simulink model "VehicleLongitudnalModel"  (R2022a)
settings: Solver=FixedStepAuto  StartTime=4192  StopTime=max(time)  FixedStep=0.01  RelTol=1e-3
values from neighbouring files (symbols this model uses):
  g = 9.81    [ModelScript.m]
  ratio_fd = ratio_fd.*0.95    [ModelScript.m]
  vehMass = 2512    [ModelScript.m]
  vehMaxPower = 400e3    (= 400000)    [ModelScript.m]
  vehTireRadius = 0.5    [ModelScript.m]
libraries: slpidlib x1
settings Model: PacingRate=0.180000  Creator=saumi  LastModifiedBy=saumilj
settings DebuggingCC: AlgebraicLoopMsg=error  ArtificialAlgebraicLoopMsg=error
settings SFSimCC: SimTargetLang=C++

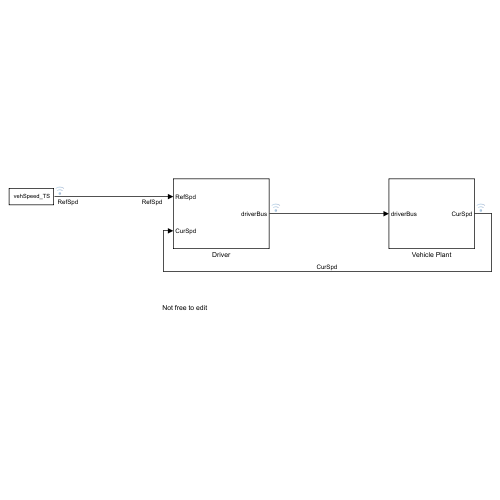
[thumbnail: Simulink's stored preview of the top-level diagram]
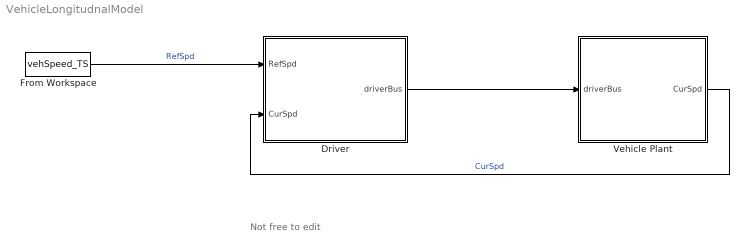
== system VehicleLongitudnalModel ==
  note: Not free to edit
  Driver : Subsystem
  From Workspace : FromWorkspace  VariableName=vehSpeed_TS
  Vehicle Plant : Subsystem
  wires:
  From Workspace/1 -> Driver/1(RefSpd)  "RefSpd"
  Vehicle Plant/1(CurSpd) -> Driver/2(CurSpd)  "CurSpd"
  Driver/1(driverBus) -> Vehicle Plant/1(driverBus)

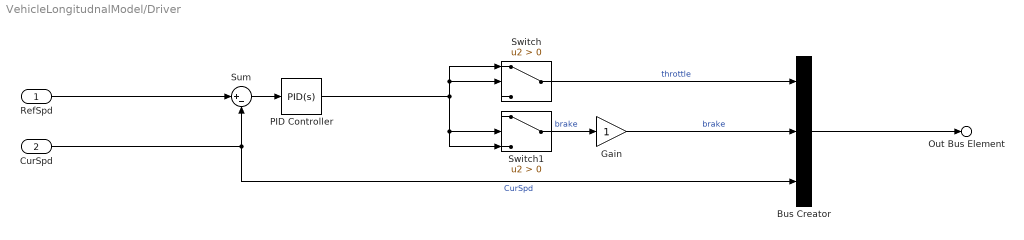
== system VehicleLongitudnalModel/Driver ==
  RefSpd : Inport
  CurSpd : Inport  Port=2
  Bus Creator : BusCreator  Inputs=3
  Gain : Gain
  PID Controller : slpidlib/PID Controller  Controller=PID  Form=Parallel  TimeDomain=Continuous-time  UseExternalTs=off  SampleTime=-1  IntegratorMethod=Forward Euler  FilterMethod=Forward Euler  ControllerParametersSource=internal  P=0.5  I=0.01  UseKiTs=off  D=0  N=100  UseFilter=on  TunerSelectOption=Transfer Function Based (PID Tuner App)  InitialConditionSource=internal  InitialConditionForIntegrator=0  InitialConditionForFilter=0  DifferentiatorICPrevScaledInput=0  ExternalReset=none  TrackingMode=off  Kt=1  LimitOutput=on  SatLimitsSource=internal  UpperSaturationLimit=1  LowerSaturationLimit=-1  LinearizeAsGain=on  AntiWindupMode=clamping  Kb=1  POutMin=[]  POutMax=[]  IOutMin=[]  IOutMax=[]  DOutMin=[]  DOutMax=[]  NOutMin=[]  NOutMax=[]  SumOutMin=[]  SumOutMax=[]  SaturationOutMin=[]  SaturationOutMax=[]  PParamMin=[]  PParamMax=[]  IParamMin=[]  IParamMax=[]  DParamMin=[]  DParamMax=[]  NParamMin=[]  NParamMax=[]  KbParamMin=[]  KbParamMax=[]  KtParamMin=[]  KtParamMax=[]  KbOutMin=[]  KbOutMax=[]  KtOutMin=[]  KtOutMax=[]  IntegratorOutMin=[]  IntegratorOutMax=[]  FilterOutMin=[]  FilterOutMax=[]  SumI1OutMin=[]  SumI1OutMax=[]  SumI2OutMin=[]  SumI2OutMax=[]  SumI3OutMin=[]  SumI3OutMax=[]  SumI4OutMin=[]  SumI4OutMax=[]  SumDOutMin=[]  SumDOutMax=[]  DifferentiatorOutMin=[]  DifferentiatorOutMax=[]  FilterDiffOutCoefMin=[]  FilterDiffOutCoefMax=[]  ReciprocalOutMin=[]  ReciprocalOutMax=[]  SumDenOutMin=[]  SumDenOutMax=[]  SumNumOutMin=[]  SumNumOutMax=[]  DivideOutMin=[]  DivideOutMax=[]  UdiffTsProdOutMin=[]  UdiffTsProdOutMax=[]  NTsProdOutMin=[]  NTsProdOutMax=[]  UintegralTsProdOutMin=[]  UintegralTsProdOutMax=[]  UngainTsProdOutMin=[]  UngainTsProdOutMax=[]  IntegratorContinuousStateAttributes=''  IntegratorStateMustResolveToSignalObject=off  IntegratorRTWStateStorageClass=Auto  FilterContinuousStateAttributes=''  FilterStateMustResolveToSignalObject=off  FilterRTWStateStorageClass=Auto  ParallelPVariant=InternalParameters  IdealPVariant=Disabled  IVariant=InternalParameters  DVariant=InternalParameters  IntegratorVariant=Continuous  SatVariant=Enabled  AWVariant=ContClampingParallel  PCopyVariant=Disabled  TRVariant=Disabled  FdbkBlocksVariant=Forward  IdealPFdbkVariant=Disabled  SatFdbkVariant=Disabled  DerivativeFilterVariant=ContFilter  NVariant=InternalParameters  NCopyVariant=Disabled  FilterICVariant=InternalICsFilter  IntegratorICVariant=InternalICs  ExternalResetVariant=Disabled  TRSumVariant=Passthrough  SumFdbkVariant=Disabled  SumVariant=Sum_PID  TsampFilterVariant=InternalTs  TsampNgainVariant=Passthrough  TsampIntegralVariant=Passthrough  ExternalSaturationOutDataTypeStr=Inherit: Same as second input  aMode=0
  Sum : Sum  Inputs=|+-
  Switch : Switch  Criteria=u2 > Threshold  SaturateOnIntegerOverflow=off  InputSameDT=off
  Switch1 : Switch  Criteria=u2 > Threshold  SaturateOnIntegerOverflow=off  InputSameDT=off
  Out Bus Element : Outport  PortName=driverBus
  wires:
  RefSpd/1 -> Sum/1
  Bus Creator/1 -> Out Bus Element/1
  CurSpd/1 -> Sum/2, Bus Creator/3  "CurSpd"
  PID Controller/1 -> Switch1/3, Switch1/2, Switch/2, Switch/1
  Switch1/1 -> Gain/1  "brake"
  Gain/1 -> Bus Creator/2  "brake"
  Switch/1 -> Bus Creator/1  "throttle"
  Sum/1 -> PID Controller/1

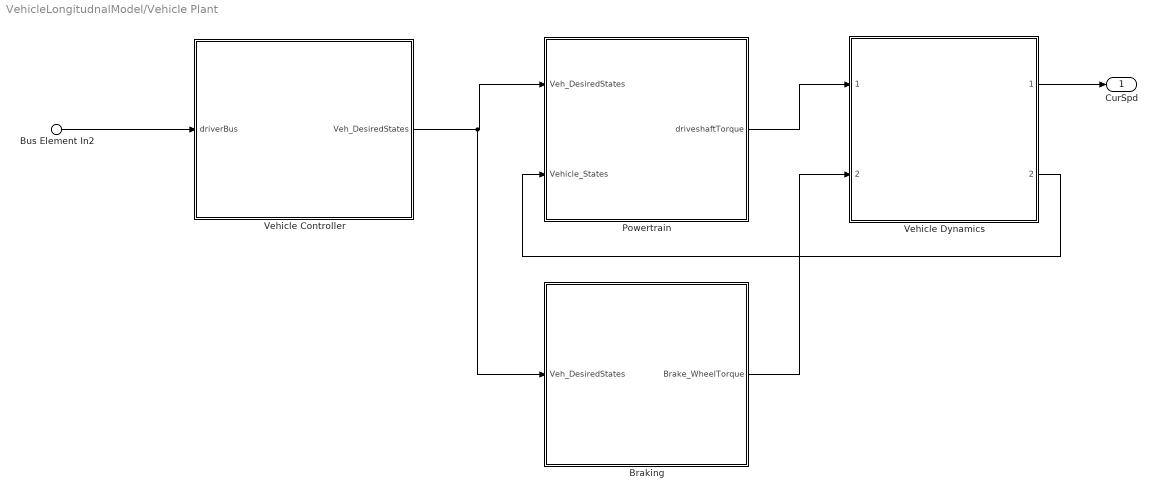
== system VehicleLongitudnalModel/Vehicle Plant ==
  Bus Element In2 : Inport  PortName=driverBus
  Braking : Subsystem
  Powertrain : Subsystem
  Vehicle Controller : Subsystem
  Vehicle Dynamics : Subsystem  ReferencedSubsystem=Vehicle_Dynamics_2
  CurSpd : Outport
  wires:
  Bus Element In2/1 -> Vehicle Controller/1(driverBus)
  Powertrain/1(driveshaftTorque) -> Vehicle Dynamics/1
  Vehicle Dynamics/1 -> CurSpd/1
  Vehicle Controller/1(Veh_DesiredStates) -> Braking/1(Veh_DesiredStates), Powertrain/1(Veh_DesiredStates)
  Vehicle Dynamics/2 -> Powertrain/2(Vehicle_States)
  Braking/1(Brake_WheelTorque) -> Vehicle Dynamics/2

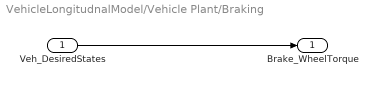
== system VehicleLongitudnalModel/Vehicle Plant/Braking ==
  Veh_DesiredStates : Inport
  Brake_WheelTorque : Outport
  wires:
  Veh_DesiredStates/1 -> Brake_WheelTorque/1

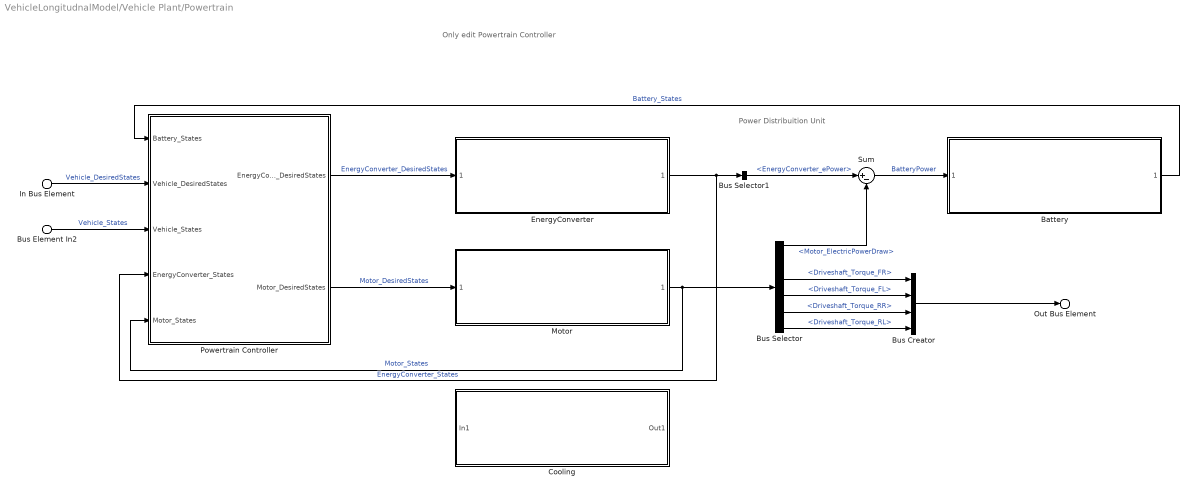
== system VehicleLongitudnalModel/Vehicle Plant/Powertrain ==
  note: Power Distribuition Unit
  note: Only edit Powertrain Controller
  In Bus Element : Inport  PortName=Veh_DesiredStates
  Bus Element In2 : Inport  Port=2  PortName=Vehicle_States
  Battery : Subsystem  ReferencedSubsystem=HV_Battery  batt_energy=64  batt_nominal_voltage=700  coolant_lpm=33.33  coolant_quantity=10  coolant_inlet_temp=25  cell_ambient_temp=35  peak_dischg_c_rate=3.8  peak_chg_c_rate=3.2  cont_dischg_c_rate=2  cont_chg_c_rate=1  peak_time=30  peak_time_dischg=0.9  batt_init_soc=0.9
  Bus Creator : BusCreator  Inputs=4
  Bus Selector : BusSelector  OutputSignals=Motor_ElectricPowerDraw,Motor_HeatGenerated,Driveshaft_Torque_FR,Driveshaft_Torque_FL,Driveshaft_Torque_RR,Driveshaft_Torque_RL
  Bus Selector1 : BusSelector  OutputSignals=EnergyConverter_ePower
  Cooling : Subsystem
  EnergyConverter : Subsystem  ReferencedSubsystem=Genset  Engine=Cummins R2.8L Tuned  Generator=Yasa P400RHC x2
  Motor : Subsystem  ReferencedSubsystem=Motor  Parameter1=YASA P400R
  Powertrain Controller : Subsystem
  Sum : Sum  Inputs=|+-
  Out Bus Element : Outport  PortName=driveshaftTorque
  wires:
  Powertrain Controller/1(EnergyConverter_DesiredStates) -> EnergyConverter/1  "EnergyConverter_DesiredStates"
  Powertrain Controller/2(Motor_DesiredStates) -> Motor/1  "Motor_DesiredStates"
  Battery/1 -> Powertrain Controller/1(Battery_States)  "Battery_States"
  Bus Selector/1 -> Sum/2  "<Motor_ElectricPowerDraw>"
  Motor/1 -> Powertrain Controller/5(Motor_States), Bus Selector/1  "Motor_States"
  Bus Creator/1 -> Out Bus Element/1
  Sum/1 -> Battery/1  "BatteryPower"
  In Bus Element/1 -> Powertrain Controller/2(Vehicle_DesiredStates)  "Vehicle_DesiredStates"
  Bus Selector/3 -> Bus Creator/1  "<Driveshaft_Torque_FR>"
  Bus Selector/4 -> Bus Creator/2  "<Driveshaft_Torque_FL>"
  Bus Selector/5 -> Bus Creator/3  "<Driveshaft_Torque_RR>"
  Bus Selector/6 -> Bus Creator/4  "<Driveshaft_Torque_RL>"
  EnergyConverter/1 -> Powertrain Controller/4(EnergyConverter_States), Bus Selector1/1  "EnergyConverter_States"
  Bus Selector1/1 -> Sum/1  "<EnergyConverter_ePower>"
  Bus Element In2/1 -> Powertrain Controller/3(Vehicle_States)  "Vehicle_States"

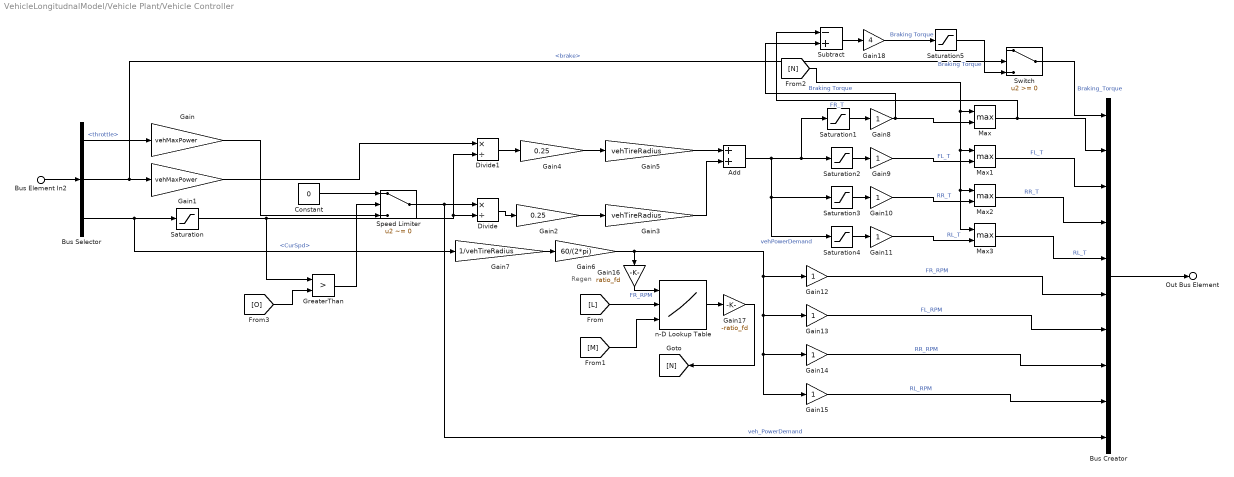
== system VehicleLongitudnalModel/Vehicle Plant/Vehicle Controller ==
  note: Regen
  Bus Element In2 : Inport  PortName=driverBus
  Add : Sum
  Bus Creator : BusCreator  Inputs=10
  Bus Selector : BusSelector  OutputSignals=throttle,brake,CurSpd
  Constant : Constant  Value=0
  Divide : Product  Inputs=*/
  Divide1 : Product  Inputs=*/
  Gain : Gain  Gain=vehMaxPower
  Gain1 : Gain  Gain=vehMaxPower
  Gain{8..15} (8 alike) : Gain
  Gain16 : Gain  Gain=ratio_fd
  Gain17 : Gain  Gain=-ratio_fd
  Gain18 : Gain  Gain=4
  Gain2 : Gain  Gain=0.25
  Gain3 : Gain  Gain=vehTireRadius
  Gain4 : Gain  Gain=0.25
  Gain5 : Gain  Gain=vehTireRadius
  Gain6 : Gain  Gain=60/(2*pi)
  Gain7 : Gain  Gain=1/vehTireRadius
  GreaterThan : RelationalOperator  Operator=>  OutDataTypeStr=boolean  RndMeth=Simplest  InputSameDT=off
  Max{,1..3} (4 alike) : MinMax  Function=max  Inputs=2
  Saturation : Saturate  UpperLimit=Inf  LowerLimit=1e-5
  Saturation{1..4} (4 alike) : Saturate  UpperLimit=vehMass.*1.*g.*vehTireRadius./4  LowerLimit=-vehMass.*1.*g.*vehTireRadius./4
  Saturation5 : Saturate  UpperLimit=0  LowerLimit=-Inf
  Speed Limiter : Switch  Criteria=u2 ~= 0  Threshold=55  SaturateOnIntegerOverflow=off  InputSameDT=off
  Subtract : Sum  Inputs=-+
  Switch : Switch  SaturateOnIntegerOverflow=off  InputSameDT=off
  n-D Lookup Table : Lookup_n-D  NumberOfTableDimensions=1  LookupTableObject=''  BreakpointsForDimension1Source=Input port  BreakpointsForDimension1=[1:2]  BreakpointsForDimension2Source=Input port  BreakpointsForDimension2=[1:2]  BreakpointsForDimension3Source=Input port  BreakpointsForDimension3=[5, 7]  BreakpointsForDimension1FirstPoint=10  BreakpointsForDimension2FirstPoint=10  BreakpointsForDimension1Spacing=12  BreakpointsForDimension2Spacing=12  IndexSearchMethod=Evenly spaced points  TableSource=Input port  Table=[4 5;16 19]  ExtrapMethod=Clip  DiagnosticForOutOfRangeInput=Warning  UseLastTableValue=on  InternalRulePriority=Speed  RndMeth=Simplest
      settings: InputPortMap=u0,p221,p5
  Out Bus Element : Outport  PortName=Veh_DesiredStates
  wires:
  Bus Element In2/1 -> Bus Selector/1
  Bus Creator/1 -> Out Bus Element/1
  Bus Selector/1 -> Gain/1  "<throttle>"
  Bus Selector/2 -> Switch/2, Gain1/1  "<brake>"
  Bus Selector/3 -> Gain7/1, Saturation/1  "<CurSpd>"
  Divide/1 -> Gain2/1
  Gain2/1 -> Gain3/1
  Gain1/1 -> Divide1/1
  Divide1/1 -> Gain4/1
  Gain4/1 -> Gain5/1
  Gain5/1 -> Add/1
  Add/1 -> Saturation1/1, Saturation2/1, Saturation4/1, Saturation3/1  "vehPowerDemand"
  Gain7/1 -> Gain6/1
  Gain6/1 -> Gain15/1, Gain14/1, Gain13/1, Gain12/1, Gain16/1
  Gain12/1 -> Bus Creator/6  "FR_RPM"
  Gain13/1 -> Bus Creator/7  "FL_RPM"
  Gain14/1 -> Bus Creator/8  "RR_RPM"
  Gain15/1 -> Bus Creator/9  "RL_RPM"
  Gain3/1 -> Add/2
  Saturation/1 -> GreaterThan/1, Divide1/2, Divide/2
  Speed Limiter/1 -> Bus Creator/10, Divide/1  "veh_PowerDemand"
  Saturation1/1 -> Gain8/1
  Saturation2/1 -> Gain9/1
  Saturation3/1 -> Gain10/1
  Saturation4/1 -> Gain11/1
  [M] -> n-D Lookup Table/3
  [L] -> n-D Lookup Table/2
  n-D Lookup Table/1 -> Gain17/1
  Gain16/1 -> n-D Lookup Table/1  "FR_RPM"
  Max/1 -> Subtract/1, Bus Creator/2  "FR_T"
  Max2/1 -> Bus Creator/4  "RR_T"
  Max3/1 -> Bus Creator/5  "RL_T"
  Max1/1 -> Bus Creator/3  "FL_T"
  Gain8/1 -> Max/2, Subtract/2  "Braking Torque"
  Gain9/1 -> Max1/2  "FL_T"
  Gain10/1 -> Max2/2  "RR_T"
  Gain11/1 -> Max3/2  "RL_T"
  Gain17/1 -> [N]
  [N] -> Max3/1, Max2/1, Max1/1, Max/1
  Subtract/1 -> Gain18/1
  Gain18/1 -> Saturation5/1  "Braking Torque"
  Saturation5/1 -> Switch/3  "Braking Torque"
  Switch/1 -> Bus Creator/1  "Braking_Torque"
  [O] -> GreaterThan/2
  GreaterThan/1 -> Speed Limiter/2
  Constant/1 -> Speed Limiter/1
  Gain/1 -> Speed Limiter/3

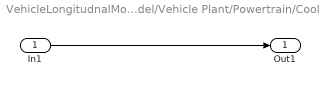
== system VehicleLongitudnalModel/Vehicle Plant/Powertrain/Cooling ==
  In1 : Inport
  Out1 : Outport
  wires:
  In1/1 -> Out1/1

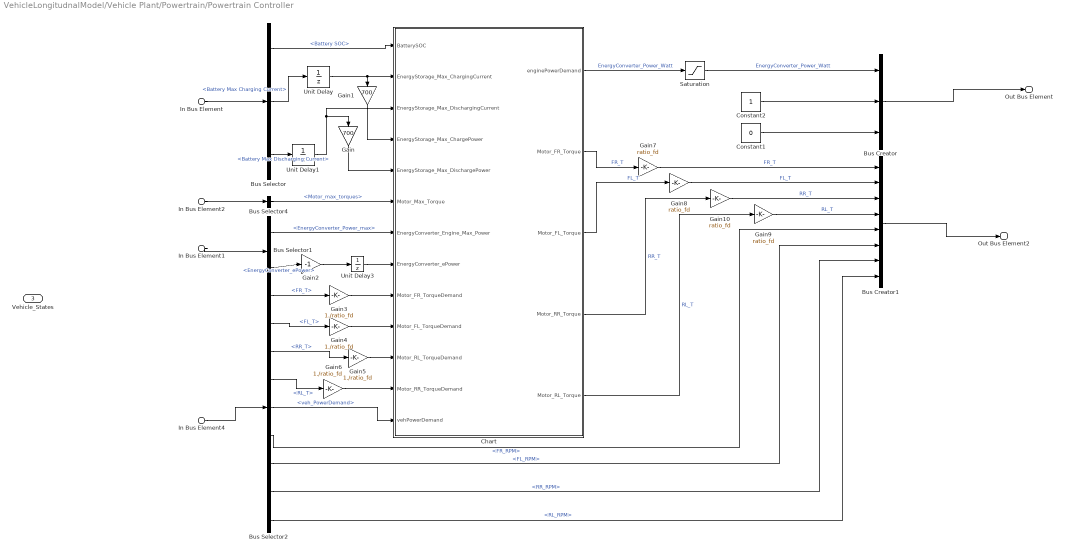
== system VehicleLongitudnalModel/Vehicle Plant/Powertrain/Powertrain Controller ==
  In Bus Element : Inport  PortName=Battery_States
  In Bus Element4 : Inport  Port=2  PortName=Vehicle_DesiredStates
  Vehicle_States : Inport  Port=3
  In Bus Element1 : Inport  Port=4  PortName=EnergyConverter_States
  In Bus Element2 : Inport  Port=5  PortName=Motor_States
  Bus Creator : BusCreator  Inputs=3
  Bus Creator1 : BusCreator  Inputs=8
  Bus Selector : BusSelector  OutputSignals=Battery SOC,Battery Max Charging Current,Battery Max Discharging Current
  Bus Selector1 : BusSelector  OutputSignals=EnergyConverter_Power_max,EnergyConverter_ePower
  Bus Selector2 : BusSelector  OutputSignals=FR_T,FL_T,RR_T,RL_T,veh_PowerDemand,FR_RPM,FL_RPM,RR_RPM,RL_RPM
  Bus Selector4 : BusSelector  OutputSignals=Motor_max_torques
  Chart : Stateflow chart  TreatAsAtomicUnit=on
      settings: PortSchema="{\"entries\":[{\"content\":{\"sides\":[{\"content\":{\"connectorIds\":[\"In1\",\"In2\",\"In3\",\"In11\",\"In12\",\"In4\",\"In5\",\"In6\",\"In7\",\"In8\",\"In9\",\"In10\",\"In13\"]},\"type\":\"ConnectorPlacement.EquallySpacedRectSide\",\"uuid\":\"78002897-e499-43f5-aefd-98a00b41a686\"},{\"content\":{\"connectorIds\":[\"Out1\",\"Out3\",\"Out2\",\"Out5\",\"Out4\"],\"side\":\"RIGHT\"},\"type\":\"ConnectorPlacement.EquallySpacedRectSide\",\"uuid\":\"e1c8cc6c-9bf6-4d66-a40e-a46d3c132e6c\"},{\"content\":{\"connectorIds\":[],\"side\":\"TOP\"},\"type\":\"ConnectorPlacement.EquallySpacedRectSide\",\"uuid\":\"d203ec9c-3185-4a9d-b862-bb67a13d539d\"}]},\"type\":\"ConnectorPlacement.EquallySpacedConnector\",\"uuid\":\"4687637b-b2d3-46f6-a39b-0e9d3f427356\"}],\"packageUris\":[\"http://schema.mathworks.com/mf0/Connector/R2020b\"],\"version\":\"1.0\"}"
  Constant1 : Constant  Value=0
  Constant2 : Constant
  Gain : Gain  Gain=700
  Gain1 : Gain  Gain=700
  Gain{7..10} (4 alike) : Gain  Gain=ratio_fd
  Gain2 : Gain  Gain=-1
  Gain{3..6} (4 alike) : Gain  Gain=1./ratio_fd
  Saturation : Saturate  UpperLimit=Inf  LowerLimit=0
  Unit Delay : UnitDelay  SampleTime=-1  HasFrameUpgradeWarning=on
  Unit Delay1 : UnitDelay  SampleTime=-1  HasFrameUpgradeWarning=on
  Unit Delay3 : UnitDelay  SampleTime=-1  HasFrameUpgradeWarning=on
  Out Bus Element : Outport  PortName=EnergyConverter_DesiredStates
  Out Bus Element2 : Outport  Port=2  PortName=Motor_DesiredStates
  wires:
  Bus Creator/1 -> Out Bus Element/1
  Chart/1(enginePowerDemand) -> Saturation/1  "EnergyConverter_Power_Watt"
  In Bus Element/1 -> Bus Selector/1
  Bus Selector/1 -> Chart/1(BatterySOC)  "<Battery SOC>"
  Saturation/1 -> Bus Creator/1  "EnergyConverter_Power_Watt"
  In Bus Element1/1 -> Bus Selector1/1
  Bus Selector1/1 -> Chart/5(EnergyConverter_Engine_Max_Power)  "<EnergyConverter_Power_max>"
  Bus Selector2/9 -> Bus Creator1/8  "<RL_RPM>"
  Bus Selector2/8 -> Bus Creator1/7  "<RR_RPM>"
  Bus Selector2/7 -> Bus Creator1/6  "<FL_RPM>"
  Bus Selector2/6 -> Bus Creator1/5  "<FR_RPM>"
  In Bus Element4/1 -> Bus Selector2/1
  In Bus Element2/1 -> Bus Selector4/1
  Bus Selector4/1 -> Chart/4(Motor_Max_Torque)  "<Motor_max_torques>"
  Bus Selector2/1 -> Gain3/1  "<FR_T>"
  Bus Selector2/2 -> Gain4/1  "<FL_T>"
  Bus Selector2/3 -> Gain5/1  "<RR_T>"
  Bus Selector2/4 -> Gain6/1  "<RL_T>"
  Bus Creator1/1 -> Out Bus Element2/1
  Chart/3(Motor_FR_Torque) -> Gain7/1  "FR_T"
  Chart/2(Motor_FL_Torque) -> Gain8/1  "FL_T"
  Chart/4(Motor_RL_Torque) -> Gain9/1  "RL_T"
  Chart/5(Motor_RR_Torque) -> Gain10/1  "RR_T"
  Bus Selector1/2 -> Gain2/1  "<EnergyConverter_ePower>"
  Unit Delay3/1 -> Chart/6(EnergyConverter_ePower)
  Bus Selector/2 -> Unit Delay/1  "<Battery Max Charging Current>"
  Bus Selector/3 -> Unit Delay1/1  "<Battery Max Discharging Current>"
  Unit Delay/1 -> Chart/2(EnergyStorage_Max_ChargingCurrent), Gain1/1
  Unit Delay1/1 -> Gain/1, Chart/3(EnergyStorage_Max_DischargingCurrent)
  Bus Selector2/5 -> Chart/13(vehPowerDemand)  "<veh_PowerDemand>"
  Gain/1 -> Chart/12(EnergyStorage_Max_DischargePower)
  Gain1/1 -> Chart/11(EnergyStorage_Max_ChargePower)
  Gain2/1 -> Unit Delay3/1
  Gain3/1 -> Chart/7(Motor_FR_TorqueDemand)
  Gain4/1 -> Chart/8(Motor_FL_TorqueDemand)
  Gain5/1 -> Chart/9(Motor_RL_TorqueDemand)
  Gain6/1 -> Chart/10(Motor_RR_TorqueDemand)
  Gain7/1 -> Bus Creator1/1  "FR_T"
  Gain8/1 -> Bus Creator1/2  "FL_T"
  Gain9/1 -> Bus Creator1/4  "RL_T"
  Gain10/1 -> Bus Creator1/3  "RR_T"
  Constant2/1 -> Bus Creator/2
  Constant1/1 -> Bus Creator/3

== stateflow chart VehicleLongitudnalModel/Vehicle Plant/Powertrain/Powertrain Controller/Chart ==
  note: batterysoc set as variables
  state REGEN_MODE
    state DEFAULT_REGEN_MODE
      Motor_FR_Torque = Motor_FR_TorqueDemand;
      Motor_FL_Torque = Motor_FL_TorqueDemand;
      Motor_RL_Torque = Motor_RL_TorqueDemand;
      Motor_RR_Torque = Motor_RR_TorqueDemand;
    state REGEN_ACTIVE_MODE
      Motor_FR_Torque = Motor_FR_TorqueDemand;
      Motor_FL_Torque = Motor_FL_TorqueDemand;
      Motor_RL_Torque = Motor_RL_TorqueDemand;
      Motor_RR_Torque = Motor_RR_TorqueDemand;
    (default) -> DEFAULT_REGEN_MODE
    DEFAULT_REGEN_MODE -> REGEN_ACTIVE_MODE : [BatterySOC<0.9]
    REGEN_ACTIVE_MODE -> DEFAULT_REGEN_MODE : [BatterySOC>=0.9]
  state DEFAULT
    %
  note: Consider Braking Torque possible as well
  state TRACTION_MODE
    state DEFAULT_MODE
      en,du:
      Motor_FR_Torque = 0;
      Motor_FL_Torque = 0;
      Motor_RL_Torque = 0;
      Motor_RR_Torque = 0;
    state MAXIMIZE_BATTERY_CHARGING
      en,du:
      switchmode =0;
      enginePowerDemand = min(max((vehPowerDemand-...
      EnergyStorage_Max_DischargePower),...
      abs(EnergyStorage_Max_ChargePower)+vehPowerDemand),...
      EnergyConverter_Engine_Max_Power);
      %Deciding motor torques
      Powertrain_Output_Power = EnergyConverter_ePower + ...
      EnergyStorage_Max_DischargePower;
      %1.2 is torque constant
      Motor_FR_Torque = min(Motor_FR_TorqueDemand,...
      Powertrain_Output_Power./700./4);
      Motor_FL_Torque = min(Motor_FR_TorqueDemand,...
      Powertrain_Output_Power./700./4);
      Motor_RR_Torque = min(Motor_FR_TorqueDemand,...
      Powertrain_Output_Power./700./4);
      Motor_RL_Torque = min(Motor_FR_TorqueDemand,...
      Powertrain_Output_Power./700./4);
      %To decide engine best BSFC or best Torque
      end
      %Torque split percentage should decide motor torques
      exit:
      switchmode = 1;
    state MAXIMIZE_BATTERY_DISCHARGING
      en,du:
      switchmode =0;
      enginePowerDemand = min(max(vehPowerDemand-...
      EnergyStorage_Max_DischargePower,...
      0),EnergyConverter_Engine_Max_Power);
      %Deciding motor torques
      Powertrain_Output_Power = EnergyConverter_ePower + ...
      EnergyStorage_Max_DischargePower;
      Motor_FR_Torque = min(Motor_FR_TorqueDemand,...
      Powertrain_Output_Power./700./4);
      Motor_FL_Torque = min(Motor_FR_TorqueDemand,...
      Powertrain_Output_Power./700./4);
      Motor_RR_Torque = min(Motor_FR_TorqueDemand,...
      Powertrain_Output_Power./700./4);
      Motor_RL_Torque = min(Motor_FR_TorqueDemand,...
      Powertrain_Output_Power./700./4);
      end
      %Torque split percentage should decide motor torques
      exit:
      switchmode =2;
    state LIMP_HOME_MODE
      en,du:
      enginePowerDemand = min(EnergyConverter_Engine_Max_Power,...
      max(vehPowerDemand,abs(EnergyStorage_Max_ChargePower)+vehPowerDemand));
      %Deciding motor torques
      Powertrain_Output_Power = EnergyConverter_ePower;
      Motor_FR_Torque = min(Motor_FR_TorqueDemand,...
      Powertrain_Output_Power./700./4);
      Motor_FL_Torque = min(Motor_FR_TorqueDemand,...
      Powertrain_Output_Power./700./4);
      Motor_RR_Torque = min(Motor_FR_TorqueDemand,...
      Powertrain_Output_Power./700./4);
      Motor_RL_Torque = min(Motor_FR_TorqueDemand,...
      Powertrain_Output_Power./700./4);
      %Torque split percentage should decide motor torques
    (default) -> DEFAULT_MODE
    DEFAULT_MODE -> MAXIMIZE_BATTERY_DISCHARGING [order 2] : [BatterySOC>=.9|switchmode ==2]
    DEFAULT_MODE -> LIMP_HOME_MODE [order 3] : [BatterySOC<=0.2]
    DEFAULT_MODE -> MAXIMIZE_BATTERY_CHARGING [order 1] : [BatterySOC<0.9 & BatterySOC>0.2 | switchmode==1]
    MAXIMIZE_BATTERY_CHARGING -> MAXIMIZE_BATTERY_DISCHARGING [order 1] : [BatterySOC>=0.9]
    MAXIMIZE_BATTERY_DISCHARGING -> MAXIMIZE_BATTERY_CHARGING : [BatterySOC<0.5]
    LIMP_HOME_MODE -> MAXIMIZE_BATTERY_CHARGING : [BatterySOC>0.2]
    MAXIMIZE_BATTERY_CHARGING -> LIMP_HOME_MODE [order 2] : [BatterySOC<=0.2]
  (default) -> DEFAULT
  DEFAULT -> REGEN_MODE [order 1] : [vehPowerDemand<0]
  DEFAULT -> TRACTION_MODE [order 2] : [vehPowerDemand>0]
  TRACTION_MODE -> REGEN_MODE : [vehPowerDemand<=0]
  REGEN_MODE -> TRACTION_MODE : [vehPowerDemand>0]
  data: BatterySOC input; EnergyStorage_Max_ChargingCurrent input; EnergyStorage_Max_DischargingCurrent input; Motor_Max_Torque input; EnergyConverter_Engine_Max_Power input; EnergyConverter_ePower input; enginePowerDemand output; Motor_FR_TorqueDemand input; Motor_FL_TorqueDemand input; Motor_RL_TorqueDemand input; Motor_RR_TorqueDemand input; EnergyStorage_Max_ChargePower input; EnergyStorage_Max_DischargePower input; vehPowerDemand input; Motor_FL_Torque output; Motor_FR_Torque output; Motor_RL_Torque output; Motor_RR_Torque output; Motor_Current local; PDU_Current local; Powertrain_Output_Power local; switchmode local =0
